simulink library "adcUtilsCh6"  (R2014a)
settings: Solver=ode45  StartTime=0.0  StopTime=10.0  RelTol=1e-3
undefined symbols (not defined in the file): angle_sensor_range, Ts, uint_range_10bit
settings Model: Creator=jrivitus  LastModifiedBy=scastro

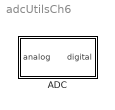
== system adcUtilsCh6 ==
  ADC : Subsystem  mask{analog_range=angle_sensor_range, digital_range=uint_range_10bit, outputType=uint16, sampleRate=Ts}
      mask prompts: analog_range "Analog range:"; digital_range "Digital range:"; outputType "Output data type:"; sampleRate "Sampling rate:"

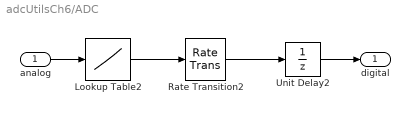
== system adcUtilsCh6/ADC ==
  analog : Inport
  Lookup Table2 : Lookup_n-D  NumberOfTableDimensions=1  BreakpointsForDimension1=analog_range  Table=digital_range  ExtrapMethod=Clip  OutDataTypeStr=outputType  InputSameDT=on
      settings: AttributesFormatString=Output data type: %<OutDataTypeStr>
  Rate Transition2 : RateTransition  Integrity=off  OutPortSampleTime=0
  Unit Delay2 : UnitDelay  SampleTime=sampleRate
  digital : Outport
  wires:
  Unit Delay2/1 -> digital/1
  analog/1 -> Lookup Table2/1
  Rate Transition2/1 -> Unit Delay2/1
  Lookup Table2/1 -> Rate Transition2/1
